simulink model "ADCS_outdated_May3"  (R2018a)
settings: Solver=VariableStepAuto  StartTime=0.0  StopTime=10.0  RelTol=1e-3
undefined symbols (not defined in the file): delta_t, GM_Earth, GM_Moon, GM_Sun, SC
settings Model: Creator=azufall  LastModifiedBy=Hridu

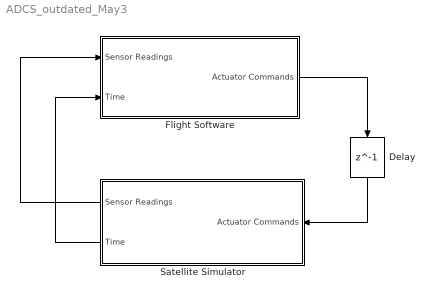
== system ADCS_outdated_May3 ==
  Delay : Delay  DelayLength=1  InitialCondition=0
  Flight Software : Subsystem
  Satellite Simulator : Subsystem
  wires:
  Flight Software/1(Actuator Commands) -> Delay/1
  Satellite Simulator/2(Time) -> Flight Software/2(Time)
  Satellite Simulator/1(Sensor Readings) -> Flight Software/1(Sensor Readings)
  Delay/1 -> Satellite Simulator/1(Actuator Commands)

== system ADCS_outdated_May3/Flight Software ==
  Sensor Readings : Inport
  Time : Inport  Port=2
  Demux : Demux  Outputs=3
  Max thrust : Gain
  Resolution Error : Rounding
  Subsystems : Subsystem
  Actuator Commands : Outport
  wires:
  Subsystems/1(RCS Command) -> Max thrust/1
  Sensor Readings/1 -> Demux/1
  Demux/1 -> Subsystems/1(Gyro)
  Demux/2 -> Subsystems/2(Sun Sensor)
  Demux/3 -> Subsystems/3(Star Tracker)
  Time/1 -> Subsystems/4(Time)
  Max thrust/1 -> Resolution Error/1
  Resolution Error/1 -> Actuator Commands/1

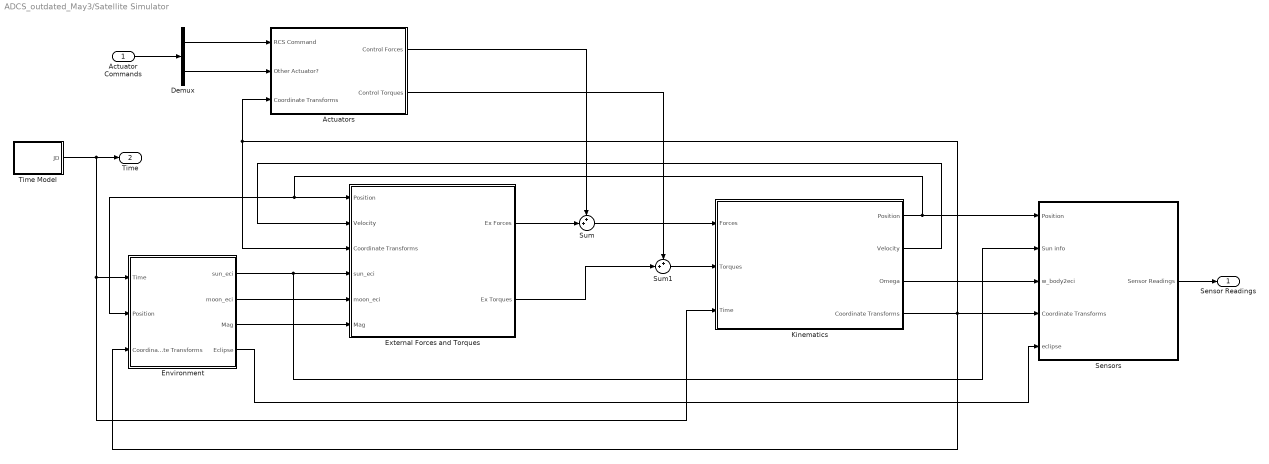
== system ADCS_outdated_May3/Satellite Simulator ==
  Actuator Commands : Inport
  Actuators : Subsystem
  Demux : Demux  Outputs=2
  Environment : Subsystem
  External Forces and Torques : Subsystem
  Kinematics : Subsystem
  Sensors : Subsystem
  Sum : Sum  Inputs=++|
  Sum1 : Sum  Inputs=++|
  Time Model : Subsystem
  Sensor Readings : Outport
  Time : Outport  Port=2
  wires:
  Actuator Commands/1 -> Demux/1
  Demux/1 -> Actuators/1(RCS Command)
  Demux/2 -> Actuators/2(Other Actuator?)
  Kinematics/3(Omega) -> Sensors/3(w_body2eci)
  Sensors/1(Sensor Readings) -> Sensor Readings/1
  Time Model/1(JD) -> Kinematics/3(Time), Environment/1(Time), Time/1
  Environment/1(sun_eci) -> Sensors/2(Sun info), External Forces and Torques/4(sun_eci)
  Environment/2(moon_eci) -> External Forces and Torques/5(moon_eci)
  Environment/3(Mag) -> External Forces and Torques/6(Mag)
  External Forces and Torques/1(Ex Forces) -> Sum/2
  Sum/1 -> Kinematics/1(Forces)
  External Forces and Torques/2(Ex Torques) -> Sum1/2
  Kinematics/2(Velocity) -> External Forces and Torques/2(Velocity)
  Kinematics/4(Coordinate Transforms) -> Environment/3(Coordinate Transforms), Actuators/3(Coordinate Transforms), External Forces and Torques/3(Coordinate Transforms), Sensors/4(Coordinate Transforms)
  Actuators/1(Control Forces) -> Sum/1
  Actuators/2(Control Torques) -> Sum1/1
  Sum1/1 -> Kinematics/2(Torques)
  Kinematics/1(Position) -> Sensors/1(Position), Environment/2(Position), External Forces and Torques/1(Position)
  Environment/4(Eclipse) -> Sensors/5(eclipse)

== system ADCS_outdated_May3/Flight Software/Subsystems ==
  Gyro : Inport
  Sun Sensor : Inport  Port=2
  Star Tracker : Inport  Port=3
  Time : Inport  Port=4
  Mode Selection : Subsystem
  RCS Controller : Subsystem
  Sensor Processing : Subsystem
  RCS Command : Outport
  wires:
  Gyro/1 -> Sensor Processing/1(Gyro_raw)
  Sun Sensor/1 -> Sensor Processing/2(Sun_raw)
  Star Tracker/1 -> Sensor Processing/3(Star_raw)
  Sensor Processing/1(Gyro_filtered) -> RCS Controller/2(Gyro), Mode Selection/1(Gyro)
  Sensor Processing/4(Eclipse) -> Mode Selection/2(Eclipse)
  Time/1 -> RCS Controller/6(Time), Mode Selection/3(Time)
  RCS Controller/1(RCS_Command) -> RCS Command/1
  Mode Selection/2(S/C Mode) -> RCS Controller/1(Mode)
  Mode Selection/1(Controller Gains) -> RCS Controller/5(Gains)
  Sensor Processing/3(Star_filtered) -> RCS Controller/4(Star)
  Sensor Processing/2(Sun_filtered) -> RCS Controller/3(Sun)

== system ADCS_outdated_May3/Satellite Simulator/Actuators ==
  RCS Command : Inport
  Other Actuator? : Inport  Port=2
  Coordinate Transforms : Inport  Port=3
  RCS Model : MATLAB Function  TreatAsAtomicUnit=on
  Control Forces : Outport
  Control Torques : Outport  Port=2
  wires:
  RCS Command/1 -> RCS Model/1(command)
  RCS Model/1(force_body) -> Control Forces/1
  RCS Model/2(torque_body) -> Control Torques/1

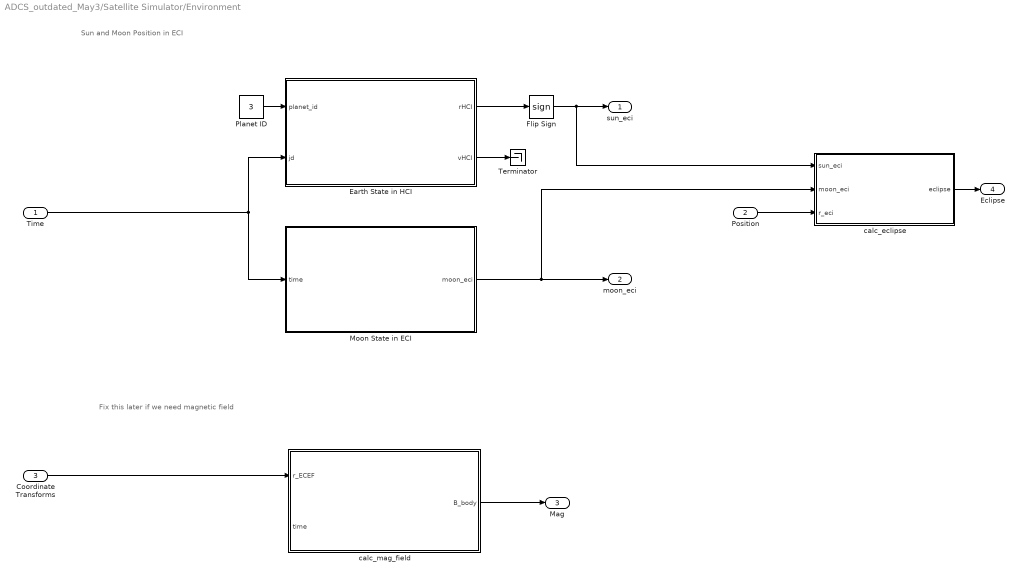
== system ADCS_outdated_May3/Satellite Simulator/Environment ==
  note: Sun and Moon Position in ECI
  note: Fix this later if we need magnetic field
  Time : Inport
  Position : Inport  Port=2
  Coordinate Transforms : Inport  Port=3
  Earth State in HCI : MATLAB Function  TreatAsAtomicUnit=on
  Flip Sign : Signum
  Moon State in ECI : MATLAB Function  TreatAsAtomicUnit=on
  Planet ID : Constant  Value=3
  Terminator : Terminator
  calc_eclipse : MATLAB Function  TreatAsAtomicUnit=on
  calc_mag_field : MATLAB Function  TreatAsAtomicUnit=on
  sun_eci : Outport
  moon_eci : Outport  Port=2
  Mag : Outport  Port=3
  Eclipse : Outport  Port=4
  wires:
  Moon State in ECI/1(moon_eci) -> calc_eclipse/2(moon_eci), moon_eci/1
  calc_mag_field/1(B_body) -> Mag/1
  calc_eclipse/1(eclipse) -> Eclipse/1
  Time/1 -> Earth State in HCI/2(jd), Moon State in ECI/1(time)
  Planet ID/1 -> Earth State in HCI/1(planet_id)
  Earth State in HCI/1(rHCI) -> Flip Sign/1
  Flip Sign/1 -> calc_eclipse/1(sun_eci), sun_eci/1
  Position/1 -> calc_eclipse/3(r_eci)
  Earth State in HCI/2(vHCI) -> Terminator/1
  Coordinate Transforms/1 -> calc_mag_field/1(r_ECEF)

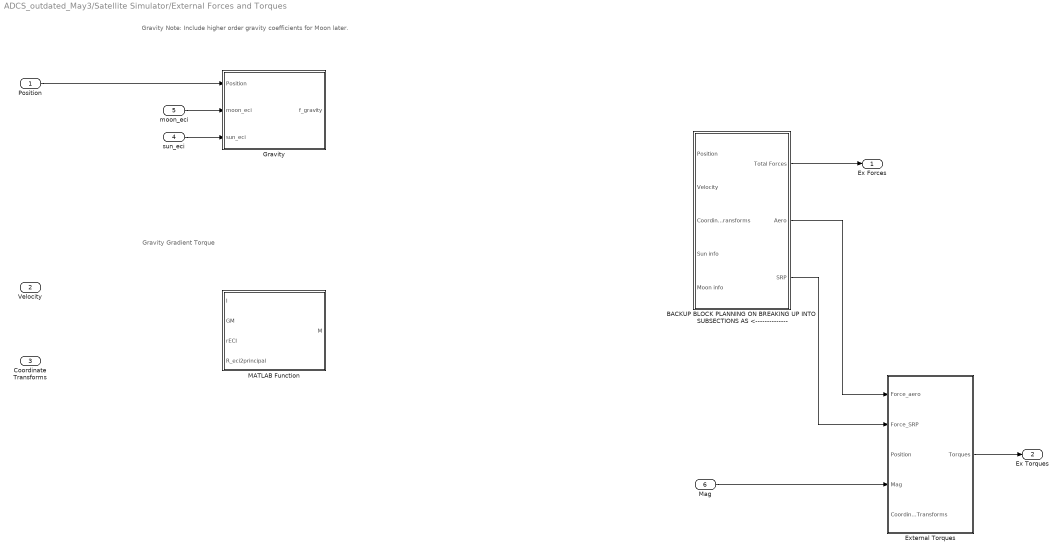
== system ADCS_outdated_May3/Satellite Simulator/External Forces and Torques ==
  note: Gravity Gradient Torque
  note: Gravity
      |
      | Note: Include higher order gravity coefficients for Moon later.
  Position : Inport
  Velocity : Inport  Port=2
  Coordinate Transforms : Inport  Port=3
  sun_eci : Inport  Port=4
  moon_eci : Inport  Port=5
  Mag : Inport  Port=6
  BACKUP BLOCK PLANNING ON BREAKING UP INTO SUBSECTIONS AS <-------------- : Subsystem
  External Torques : Subsystem
  Gravity : Subsystem
  MATLAB Function : MATLAB Function  TreatAsAtomicUnit=on
  Ex Forces : Outport
  Ex Torques : Outport  Port=2
  wires:
  Mag/1 -> External Torques/4(Mag)
  BACKUP BLOCK PLANNING ON BREAKING UP INTO SUBSECTIONS AS <--------------/1(Total Forces) -> Ex Forces/1
  External Torques/1(Torques) -> Ex Torques/1
  BACKUP BLOCK PLANNING ON BREAKING UP INTO SUBSECTIONS AS <--------------/2(Aero) -> External Torques/1(Force_aero)
  BACKUP BLOCK PLANNING ON BREAKING UP INTO SUBSECTIONS AS <--------------/3(SRP) -> External Torques/2(Force_SRP)
  Position/1 -> Gravity/1(Position)
  moon_eci/1 -> Gravity/2(moon_eci)
  sun_eci/1 -> Gravity/3(sun_eci)

== system ADCS_outdated_May3/Satellite Simulator/Kinematics ==
  Forces : Inport
  Torques : Inport  Port=2
  Time : Inport  Port=3
  Calc Coordinate Transforms : Subsystem
  Position Kinematics : Subsystem
  Rotation Kinematics : Subsystem
  TEST POSITION KINEMATICS : Subsystem
  Position : Outport
  Velocity : Outport  Port=2
  Omega : Outport  Port=3
  Coordinate Transforms : Outport  Port=4
  wires:
  Forces/1 -> Position Kinematics/1(a_eci)
  Torques/1 -> Rotation Kinematics/1(tor)
  Rotation Kinematics/2(w) -> Omega/1
  Rotation Kinematics/1(q) -> Calc Coordinate Transforms/4(Attitude)
  Position Kinematics/1(r_eci) -> Position/1, Calc Coordinate Transforms/1(Position)
  Position Kinematics/2(v_eci) -> Velocity/1, Calc Coordinate Transforms/2(Velocity)
  Calc Coordinate Transforms/1(Coordinate Transforms) -> Coordinate Transforms/1
  Time/1 -> Calc Coordinate Transforms/3(Time)

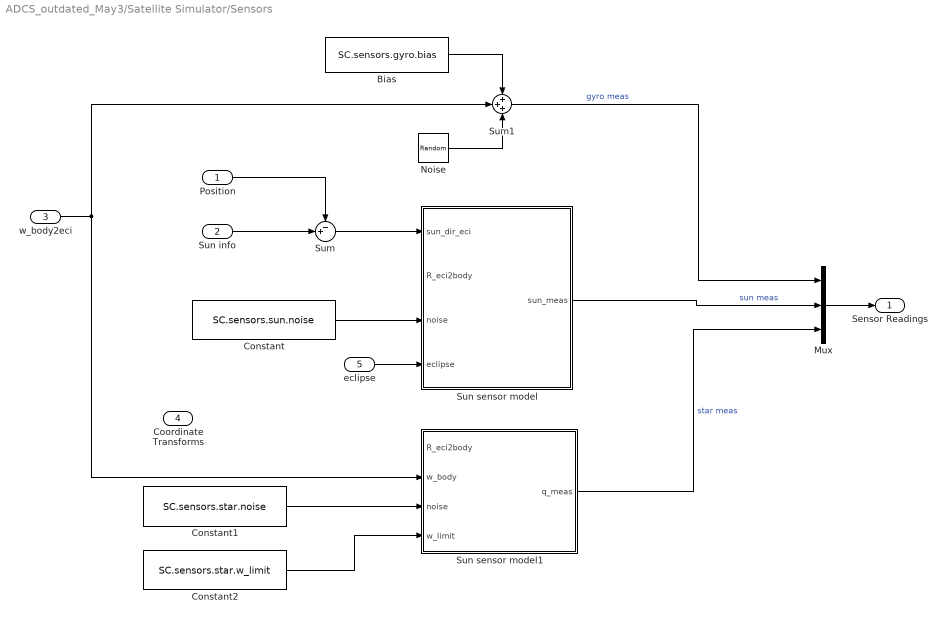
== system ADCS_outdated_May3/Satellite Simulator/Sensors ==
  Position : Inport
  Sun info : Inport  Port=2
  w_body2eci : Inport  Port=3
  Coordinate Transforms : Inport  Port=4
  eclipse : Inport  Port=5
  Bias : Constant  Value=SC.sensors.gyro.bias
  Constant : Constant  Value=SC.sensors.sun.noise
  Constant1 : Constant  Value=SC.sensors.star.noise
  Constant2 : Constant  Value=SC.sensors.star.w_limit
  Mux : Mux  Inputs=3
  Noise : RandomNumber  Variance=SC.sensors.gyro.noise  SampleTime=0.1
  Sum : Sum  Inputs=-+|
  Sum1 : Sum  Inputs=+++
  Sun sensor model : MATLAB Function  TreatAsAtomicUnit=on
  Sun sensor model1 : MATLAB Function  TreatAsAtomicUnit=on
  Sensor Readings : Outport
  wires:
  Mux/1 -> Sensor Readings/1
  Sun sensor model1/1(q_meas) -> Mux/3  "star meas"
  Sun info/1 -> Sum/2
  Position/1 -> Sum/1
  Constant/1 -> Sun sensor model/3(noise)
  Sum/1 -> Sun sensor model/1(sun_dir_eci)
  Sun sensor model/1(sun_meas) -> Mux/2  "sun meas"
  Noise/1 -> Sum1/3
  Bias/1 -> Sum1/1
  w_body2eci/1 -> Sun sensor model1/2(w_body), Sum1/2
  Sum1/1 -> Mux/1  "gyro meas"
  Constant1/1 -> Sun sensor model1/3(noise)
  Constant2/1 -> Sun sensor model1/4(w_limit)
  eclipse/1 -> Sun sensor model/4(eclipse)

== system ADCS_outdated_May3/Satellite Simulator/Time Model ==
  Constant : Constant  Value=SC.initial_state.date  VectorParams1D=off
  Constant1 : Constant  Value=delta_t
  Date2JD : MATLAB Function  TreatAsAtomicUnit=on
  Delay : Delay  DelayLength=1  InitialConditionSource=Input port  InitialCondition=0
      settings: InputPortMap=u0,p4
  Sum : Sum  Inputs=|++
  JD : Outport
  wires:
  Sum/1 -> JD/1, Delay/1
  Constant1/1 -> Sum/2
  Delay/1 -> Sum/1
  Constant/1 -> Date2JD/1(date)
  Date2JD/1(JD) -> Delay/2

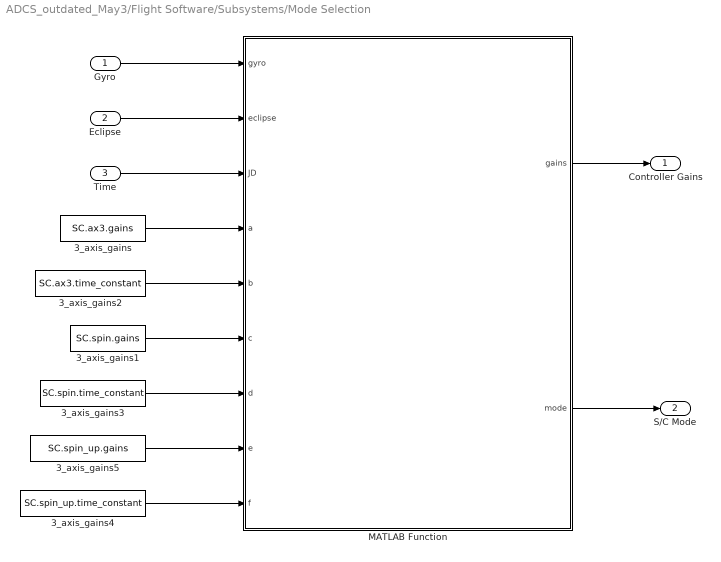
== system ADCS_outdated_May3/Flight Software/Subsystems/Mode Selection ==
  Gyro : Inport
  Eclipse : Inport  Port=2
  Time : Inport  Port=3
  3_axis_gains : Constant  Value=SC.ax3.gains
  3_axis_gains1 : Constant  Value=SC.spin.gains
  3_axis_gains2 : Constant  Value=SC.ax3.time_constant
  3_axis_gains3 : Constant  Value=SC.spin.time_constant
  3_axis_gains4 : Constant  Value=SC.spin_up.time_constant
  3_axis_gains5 : Constant  Value=SC.spin_up.gains
  MATLAB Function : MATLAB Function  TreatAsAtomicUnit=on
  Controller Gains : Outport
  S/C Mode : Outport  Port=2
  wires:
  Time/1 -> MATLAB Function/3(JD)
  Gyro/1 -> MATLAB Function/1(gyro)
  Eclipse/1 -> MATLAB Function/2(eclipse)
  MATLAB Function/1(gains) -> Controller Gains/1
  MATLAB Function/2(mode) -> S/C Mode/1
  3_axis_gains/1 -> MATLAB Function/4(a)
  3_axis_gains2/1 -> MATLAB Function/5(b)
  3_axis_gains1/1 -> MATLAB Function/6(c)
  3_axis_gains3/1 -> MATLAB Function/7(d)
  3_axis_gains5/1 -> MATLAB Function/8(e)
  3_axis_gains4/1 -> MATLAB Function/9(f)

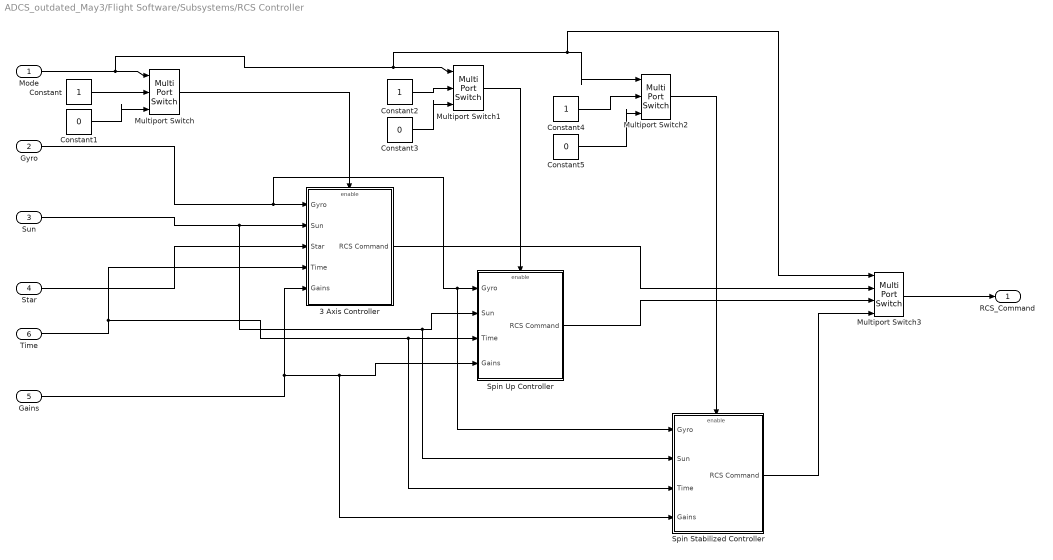
== system ADCS_outdated_May3/Flight Software/Subsystems/RCS Controller ==
  Mode : Inport
  Gyro : Inport  Port=2
  Sun : Inport  Port=3
  Star : Inport  Port=4
  Gains : Inport  Port=5
  Time : Inport  Port=6
  3 Axis Controller : Subsystem  TreatAsAtomicUnit=on
  Constant : Constant
  Constant1 : Constant  Value=0
  Constant2 : Constant
  Constant3 : Constant  Value=0
  Constant4 : Constant
  Constant5 : Constant  Value=0
  Multiport Switch : MultiPortSwitch  Inputs=2
  Multiport Switch1 : MultiPortSwitch  Inputs=2
  Multiport Switch2 : MultiPortSwitch  Inputs=2
  Multiport Switch3 : MultiPortSwitch
  Spin Stabilized Controller : Subsystem  TreatAsAtomicUnit=on
  Spin Up Controller : Subsystem  TreatAsAtomicUnit=on
  RCS_Command : Outport
  wires:
  Multiport Switch/1 -> 3 Axis Controller/Enable
  Multiport Switch1/1 -> Spin Up Controller/Enable
  Multiport Switch2/1 -> Spin Stabilized Controller/Enable
  Mode/1 -> Multiport Switch3/1, Multiport Switch2/1, Multiport Switch1/1, Multiport Switch/1
  Gyro/1 -> Spin Stabilized Controller/1(Gyro), Spin Up Controller/1(Gyro), 3 Axis Controller/1(Gyro)
  Sun/1 -> Spin Stabilized Controller/2(Sun), Spin Up Controller/2(Sun), 3 Axis Controller/2(Sun)
  Star/1 -> 3 Axis Controller/3(Star)
  Time/1 -> Spin Stabilized Controller/3(Time), Spin Up Controller/3(Time), 3 Axis Controller/4(Time)
  Gains/1 -> Spin Stabilized Controller/4(Gains), Spin Up Controller/4(Gains), 3 Axis Controller/5(Gains)
  3 Axis Controller/1(RCS Command) -> Multiport Switch3/2
  Spin Up Controller/1(RCS Command) -> Multiport Switch3/3
  Spin Stabilized Controller/1(RCS Command) -> Multiport Switch3/4
  Multiport Switch3/1 -> RCS_Command/1
  Constant/1 -> Multiport Switch/2
  Constant1/1 -> Multiport Switch/3
  Constant2/1 -> Multiport Switch1/2
  Constant3/1 -> Multiport Switch1/3
  Constant4/1 -> Multiport Switch2/2
  Constant5/1 -> Multiport Switch2/3

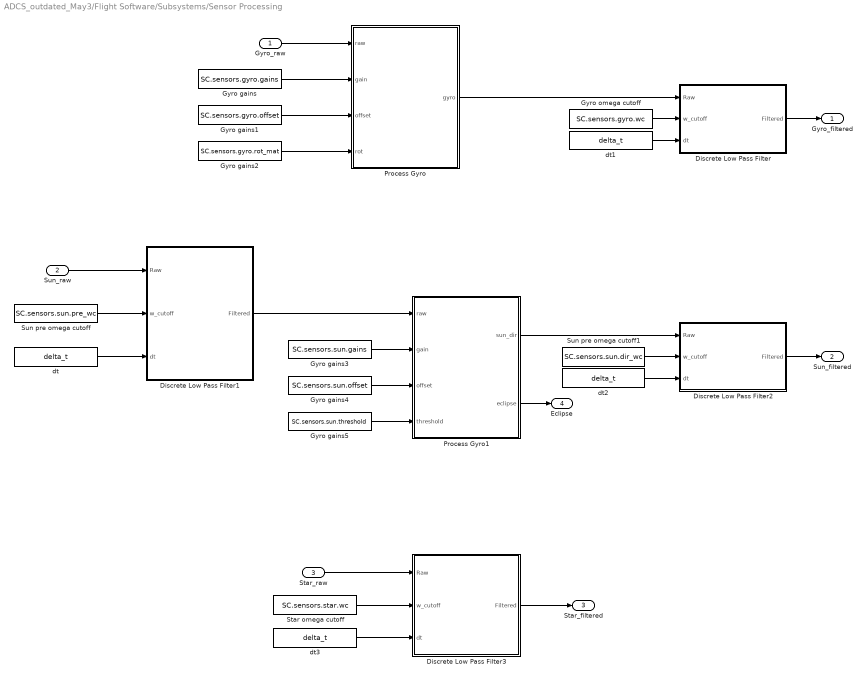
== system ADCS_outdated_May3/Flight Software/Subsystems/Sensor Processing ==
  Gyro_raw : Inport
  Sun_raw : Inport  Port=2
  Star_raw : Inport  Port=3
  Discrete Low Pass Filter : Subsystem
  Discrete Low Pass Filter1 : Subsystem
  Discrete Low Pass Filter2 : Subsystem
  Discrete Low Pass Filter3 : Subsystem
  Gyro gains : Constant  Value=SC.sensors.gyro.gains
  Gyro gains1 : Constant  Value=SC.sensors.gyro.offset
  Gyro gains2 : Constant  Value=SC.sensors.gyro.rot_mat
  Gyro gains3 : Constant  Value=SC.sensors.sun.gains
  Gyro gains4 : Constant  Value=SC.sensors.sun.offset
  Gyro gains5 : Constant  Value=SC.sensors.sun.threshold
  Gyro omega cutoff : Constant  Value=SC.sensors.gyro.wc
  Process Gyro : MATLAB Function  TreatAsAtomicUnit=on
  Process Gyro1 : MATLAB Function  TreatAsAtomicUnit=on
  Star omega cutoff : Constant  Value=SC.sensors.star.wc
  Sun pre omega cutoff : Constant  Value=SC.sensors.sun.pre_wc
  Sun pre omega cutoff1 : Constant  Value=SC.sensors.sun.dir_wc
  dt{,1..3} (4 alike) : Constant  Value=delta_t
  Gyro_filtered : Outport
  Sun_filtered : Outport  Port=2
  Star_filtered : Outport  Port=3
  Eclipse : Outport  Port=4
  wires:
  Gyro_raw/1 -> Process Gyro/1(raw)
  Gyro gains/1 -> Process Gyro/2(gain)
  Gyro gains1/1 -> Process Gyro/3(offset)
  Gyro gains2/1 -> Process Gyro/4(rot)
  Discrete Low Pass Filter/1(Filtered) -> Gyro_filtered/1
  Process Gyro/1(gyro) -> Discrete Low Pass Filter/1(Raw)
  Gyro omega cutoff/1 -> Discrete Low Pass Filter/2(w_cutoff)
  dt1/1 -> Discrete Low Pass Filter/3(dt)
  Sun_raw/1 -> Discrete Low Pass Filter1/1(Raw)
  Discrete Low Pass Filter1/1(Filtered) -> Process Gyro1/1(raw)
  Discrete Low Pass Filter2/1(Filtered) -> Sun_filtered/1
  Process Gyro1/1(sun_dir) -> Discrete Low Pass Filter2/1(Raw)
  Process Gyro1/2(eclipse) -> Eclipse/1
  Sun pre omega cutoff/1 -> Discrete Low Pass Filter1/2(w_cutoff)
  dt/1 -> Discrete Low Pass Filter1/3(dt)
  Gyro gains3/1 -> Process Gyro1/2(gain)
  Gyro gains4/1 -> Process Gyro1/3(offset)
  Gyro gains5/1 -> Process Gyro1/4(threshold)
  Sun pre omega cutoff1/1 -> Discrete Low Pass Filter2/2(w_cutoff)
  dt2/1 -> Discrete Low Pass Filter2/3(dt)
  Star_raw/1 -> Discrete Low Pass Filter3/1(Raw)
  Discrete Low Pass Filter3/1(Filtered) -> Star_filtered/1
  Star omega cutoff/1 -> Discrete Low Pass Filter3/2(w_cutoff)
  dt3/1 -> Discrete Low Pass Filter3/3(dt)

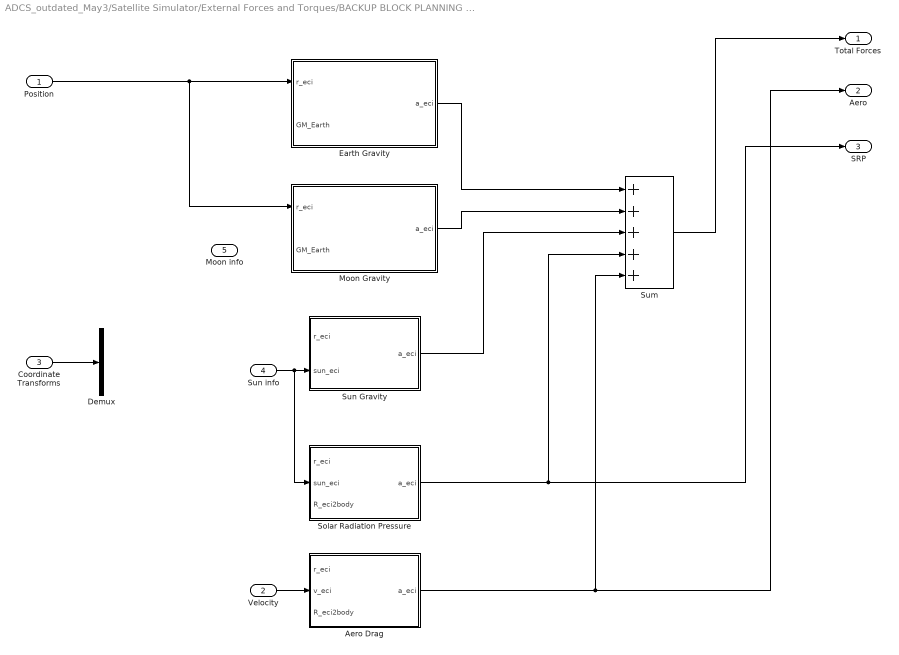
== system ADCS_outdated_May3/Satellite Simulator/External Forces and Torques/BACKUP BLOCK PLANNING ON BREAKING UP INTO SUBSECTIONS AS <-------------- ==
  Position : Inport
  Velocity : Inport  Port=2
  Coordinate Transforms : Inport  Port=3
  Sun info : Inport  Port=4
  Moon info : Inport  Port=5
  Aero Drag : MATLAB Function  TreatAsAtomicUnit=on
  Demux : Demux
  Earth Gravity : MATLAB Function  TreatAsAtomicUnit=on
  Moon Gravity : MATLAB Function  TreatAsAtomicUnit=on
  Solar Radiation Pressure : MATLAB Function  TreatAsAtomicUnit=on
  Sum : Sum  Inputs=+++++
  Sun Gravity : MATLAB Function  TreatAsAtomicUnit=on
  Total Forces : Outport
  Aero : Outport  Port=2
  SRP : Outport  Port=3
  wires:
  Position/1 -> Moon Gravity/1(r_eci), Earth Gravity/1(r_eci)
  Sun info/1 -> Solar Radiation Pressure/2(sun_eci), Sun Gravity/2(sun_eci)
  Solar Radiation Pressure/1(a_eci) -> Sum/4, SRP/1
  Aero Drag/1(a_eci) -> Sum/5, Aero/1
  Sum/1 -> Total Forces/1
  Earth Gravity/1(a_eci) -> Sum/1
  Sun Gravity/1(a_eci) -> Sum/3
  Velocity/1 -> Aero Drag/2(v_eci)
  Coordinate Transforms/1 -> Demux/1
  Moon Gravity/1(a_eci) -> Sum/2

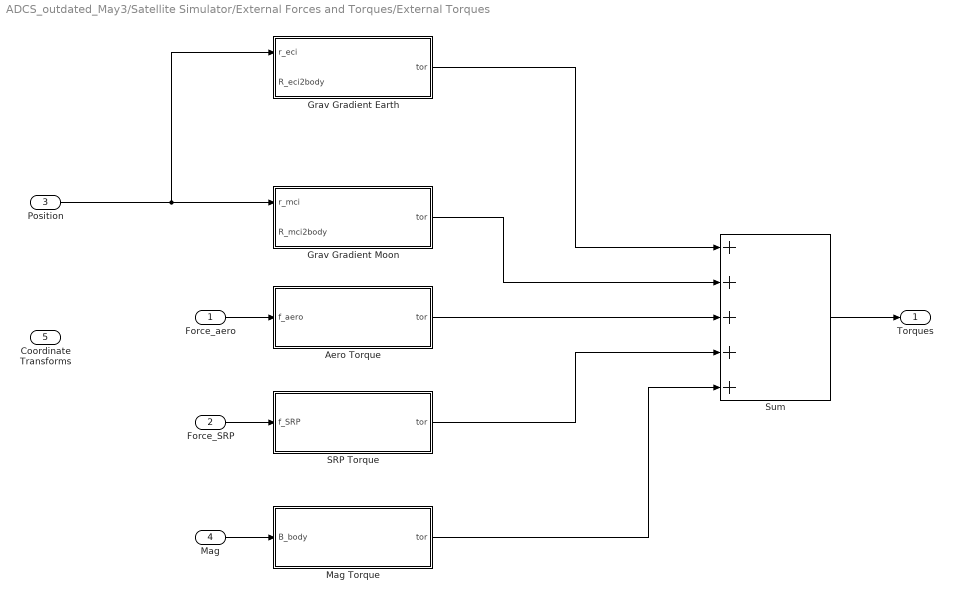
== system ADCS_outdated_May3/Satellite Simulator/External Forces and Torques/External Torques ==
  Force_aero : Inport
  Force_SRP : Inport  Port=2
  Position : Inport  Port=3
  Mag : Inport  Port=4
  Coordinate Transforms : Inport  Port=5
  Aero Torque : MATLAB Function  TreatAsAtomicUnit=on
  Grav Gradient Earth : MATLAB Function  TreatAsAtomicUnit=on
  Grav Gradient Moon : MATLAB Function  TreatAsAtomicUnit=on
  Mag Torque : MATLAB Function  TreatAsAtomicUnit=on
  SRP Torque : MATLAB Function  TreatAsAtomicUnit=on
  Sum : Sum  Inputs=5
  Torques : Outport
  wires:
  Position/1 -> Grav Gradient Moon/1(r_mci), Grav Gradient Earth/1(r_eci)
  Sum/1 -> Torques/1
  Grav Gradient Earth/1(tor) -> Sum/1
  Grav Gradient Moon/1(tor) -> Sum/2
  Aero Torque/1(tor) -> Sum/3
  Force_aero/1 -> Aero Torque/1(f_aero)
  Force_SRP/1 -> SRP Torque/1(f_SRP)
  SRP Torque/1(tor) -> Sum/4
  Mag Torque/1(tor) -> Sum/5
  Mag/1 -> Mag Torque/1(B_body)

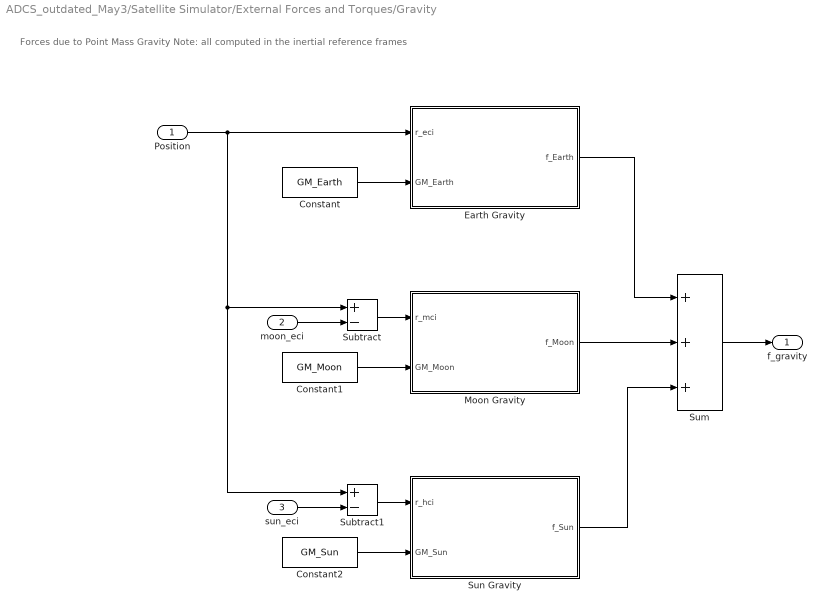
== system ADCS_outdated_May3/Satellite Simulator/External Forces and Torques/Gravity ==
  note: Forces due to Point Mass Gravity
      |
      | Note: all computed in the inertial reference frames
  Position : Inport
  moon_eci : Inport  Port=2
  sun_eci : Inport  Port=3
  Constant : Constant  Value=GM_Earth
  Constant1 : Constant  Value=GM_Moon
  Constant2 : Constant  Value=GM_Sun
  Earth Gravity : MATLAB Function  TreatAsAtomicUnit=on
  Moon Gravity : MATLAB Function  TreatAsAtomicUnit=on
  Subtract : Sum  Inputs=+-
  Subtract1 : Sum  Inputs=+-
  Sum : Sum  Inputs=+++
  Sun Gravity : MATLAB Function  TreatAsAtomicUnit=on
  f_gravity : Outport
  wires:
  Position/1 -> Earth Gravity/1(r_eci), Subtract/1, Subtract1/1
  Sum/1 -> f_gravity/1
  Earth Gravity/1(f_Earth) -> Sum/1
  Sun Gravity/1(f_Sun) -> Sum/3
  Moon Gravity/1(f_Moon) -> Sum/2
  moon_eci/1 -> Subtract/2
  Subtract/1 -> Moon Gravity/1(r_mci)
  Subtract1/1 -> Sun Gravity/1(r_hci)
  sun_eci/1 -> Subtract1/2
  Constant/1 -> Earth Gravity/2(GM_Earth)
  Constant1/1 -> Moon Gravity/2(GM_Moon)
  Constant2/1 -> Sun Gravity/2(GM_Sun)

== system ADCS_outdated_May3/Satellite Simulator/Kinematics/Calc Coordinate Transforms ==
  Position : Inport
  Velocity : Inport  Port=2
  Time : Inport  Port=3
  Attitude : Inport  Port=4
  Mux : Mux
  Coordinate Transforms : Outport
  wires:
  Mux/1 -> Coordinate Transforms/1

== system ADCS_outdated_May3/Satellite Simulator/Kinematics/Position Kinematics ==
  a_eci : Inport
  3 DOF Kinematics : MATLAB Function  TreatAsAtomicUnit=on
  Constant : Constant  Value=SC.initial_state.r_eci
  Constant1 : Constant  Value=SC.initial_state.v_eci
  Constant2 : Constant  Value=delta_t
  Delay : Delay  DelayLength=1  InitialConditionSource=Input port  InitialCondition=0
      settings: InputPortMap=u0,p4
  Delay1 : Delay  DelayLength=1  InitialConditionSource=Input port  InitialCondition=0
      settings: InputPortMap=u0,p4
  r_eci : Outport
  v_eci : Outport  Port=2
  wires:
  a_eci/1 -> 3 DOF Kinematics/3(a_eci)
  3 DOF Kinematics/1(r_eci) -> Delay/1, r_eci/1
  3 DOF Kinematics/2(v_eci) -> Delay1/1, v_eci/1
  Delay/1 -> 3 DOF Kinematics/1(r_eci_i)
  Delay1/1 -> 3 DOF Kinematics/2(v_eci_i)
  Constant/1 -> Delay/2
  Constant1/1 -> Delay1/2
  Constant2/1 -> 3 DOF Kinematics/4(dt)

== system ADCS_outdated_May3/Satellite Simulator/Kinematics/Rotation Kinematics ==
  tor : Inport
  Constant : Constant  Value=SC.initial_state.q
  Constant1 : Constant  Value=SC.initial_state.w
  Constant2 : Constant  Value=delta_t
  Delay : Delay  DelayLength=1  InitialConditionSource=Input port  InitialCondition=0
      settings: InputPortMap=u0,p4
  Delay1 : Delay  DelayLength=1  InitialConditionSource=Input port  InitialCondition=0
      settings: InputPortMap=u0,p4
  Euler Equations : MATLAB Function  TreatAsAtomicUnit=on
  q : Outport
  w : Outport  Port=2
  wires:
  tor/1 -> Euler Equations/3(tor)
  Euler Equations/1(q) -> Delay/1, q/1
  Delay/1 -> Euler Equations/1(q_i)
  Delay1/1 -> Euler Equations/2(w_i)
  Constant/1 -> Delay/2
  Constant1/1 -> Delay1/2
  Constant2/1 -> Euler Equations/4(dt)
  Euler Equations/2(w) -> Delay1/1, w/1

== system ADCS_outdated_May3/Satellite Simulator/Kinematics/TEST POSITION KINEMATICS ==
  a_eci : Inport
  Constant3 : Constant  Value=SC.initial_state.r_eci
  Constant4 : Constant  Value=SC.initial_state.v_eci
  Integrator : Integrator  InitialConditionSource=external
  Integrator1 : Integrator  InitialConditionSource=external
  r_eci : Outport
  v_eci : Outport  Port=2
  wires:
  Constant4/1 -> Integrator/2
  a_eci/1 -> Integrator/1
  Integrator/1 -> v_eci/1, Integrator1/1
  Constant3/1 -> Integrator1/2
  Integrator1/1 -> r_eci/1

== system ADCS_outdated_May3/Flight Software/Subsystems/RCS Controller/3 Axis Controller ==
  Gyro : Inport
  Sun : Inport  Port=2
  Star : Inport  Port=3
  Time : Inport  Port=4
  Gains : Inport  Port=5
  Enable : EnablePort
  RCS Command : Outport
  wires:
  Gyro/1 -> RCS Command/1

== system ADCS_outdated_May3/Flight Software/Subsystems/RCS Controller/Spin Stabilized Controller ==
  Gyro : Inport
  Sun : Inport  Port=2
  Time : Inport  Port=3
  Gains : Inport  Port=4
  Enable : EnablePort
  RCS Command : Outport
  wires:
  Gyro/1 -> RCS Command/1

== system ADCS_outdated_May3/Flight Software/Subsystems/RCS Controller/Spin Up Controller ==
  Gyro : Inport
  Sun : Inport  Port=2
  Time : Inport  Port=3
  Gains : Inport  Port=4
  Enable : EnablePort
  RCS Command : Outport
  wires:
  Gyro/1 -> RCS Command/1

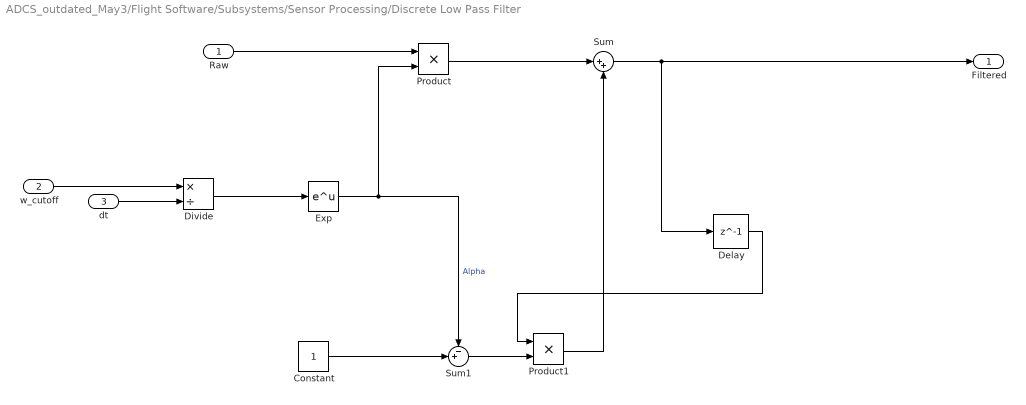
== system ADCS_outdated_May3/Flight Software/Subsystems/Sensor Processing/Discrete Low Pass Filter ==
  Raw : Inport
  w_cutoff : Inport  Port=2
  dt : Inport  Port=3
  Constant : Constant
  Delay : Delay  DelayLength=1  InitialCondition=0
  Divide : Product  Inputs=*/
  Exp : Math  SaturateOnIntegerOverflow=on
  Product : Product
  Product1 : Product
  Sum : Sum  Inputs=|++
  Sum1 : Sum  Inputs=-+|
  Filtered : Outport
  wires:
  w_cutoff/1 -> Divide/1
  dt/1 -> Divide/2
  Divide/1 -> Exp/1
  Exp/1 -> Sum1/1, Product/2  "Alpha"
  Raw/1 -> Product/1
  Product/1 -> Sum/1
  Sum/1 -> Delay/1, Filtered/1
  Constant/1 -> Sum1/2
  Sum1/1 -> Product1/2
  Delay/1 -> Product1/1
  Product1/1 -> Sum/2

== system ADCS_outdated_May3/Flight Software/Subsystems/Sensor Processing/Discrete Low Pass Filter1 ==
  Raw : Inport
  w_cutoff : Inport  Port=2
  dt : Inport  Port=3
  Constant : Constant
  Delay : Delay  DelayLength=1  InitialCondition=0
  Divide : Product  Inputs=*/
  Exp : Math  SaturateOnIntegerOverflow=on
  Product : Product
  Product1 : Product
  Sum : Sum  Inputs=|++
  Sum1 : Sum  Inputs=-+|
  Filtered : Outport
  wires:
  w_cutoff/1 -> Divide/1
  dt/1 -> Divide/2
  Divide/1 -> Exp/1
  Exp/1 -> Sum1/1, Product/2  "Alpha"
  Raw/1 -> Product/1
  Product/1 -> Sum/1
  Sum/1 -> Delay/1, Filtered/1
  Constant/1 -> Sum1/2
  Sum1/1 -> Product1/2
  Delay/1 -> Product1/1
  Product1/1 -> Sum/2

== system ADCS_outdated_May3/Flight Software/Subsystems/Sensor Processing/Discrete Low Pass Filter2 ==
  Raw : Inport
  w_cutoff : Inport  Port=2
  dt : Inport  Port=3
  Constant : Constant
  Delay : Delay  DelayLength=1  InitialCondition=0
  Divide : Product  Inputs=*/
  Exp : Math  SaturateOnIntegerOverflow=on
  Product : Product
  Product1 : Product
  Sum : Sum  Inputs=|++
  Sum1 : Sum  Inputs=-+|
  Filtered : Outport
  wires:
  w_cutoff/1 -> Divide/1
  dt/1 -> Divide/2
  Divide/1 -> Exp/1
  Exp/1 -> Sum1/1, Product/2  "Alpha"
  Raw/1 -> Product/1
  Product/1 -> Sum/1
  Sum/1 -> Delay/1, Filtered/1
  Constant/1 -> Sum1/2
  Sum1/1 -> Product1/2
  Delay/1 -> Product1/1
  Product1/1 -> Sum/2

== system ADCS_outdated_May3/Flight Software/Subsystems/Sensor Processing/Discrete Low Pass Filter3 ==
  Raw : Inport
  w_cutoff : Inport  Port=2
  dt : Inport  Port=3
  Constant : Constant
  Delay : Delay  DelayLength=1  InitialCondition=0
  Divide : Product  Inputs=*/
  Exp : Math  SaturateOnIntegerOverflow=on
  Product : Product
  Product1 : Product
  Sum : Sum  Inputs=|++
  Sum1 : Sum  Inputs=-+|
  Filtered : Outport
  wires:
  w_cutoff/1 -> Divide/1
  dt/1 -> Divide/2
  Divide/1 -> Exp/1
  Exp/1 -> Sum1/1, Product/2  "Alpha"
  Raw/1 -> Product/1
  Product/1 -> Sum/1
  Sum/1 -> Delay/1, Filtered/1
  Constant/1 -> Sum1/2
  Sum1/1 -> Product1/2
  Delay/1 -> Product1/1
  Product1/1 -> Sum/2

== matlab function ADCS_outdated_May3/Flight Software/Subsystems/Sensor Processing/Process Gyro ==
  data: raw input; gyro output; gain input; offset input; rot input
function gyro = process_gyro(raw, gain, offset, rot)

temp = rot * raw;
gyro = gain * (temp - offset);

== matlab function ADCS_outdated_May3/Flight Software/Subsystems/Mode Selection/MATLAB Function ==
  data: gyro input; gains output; eclipse input; JD input; mode output; a input; b input; c input; d input; e input; f input
function [gains, mode]  = Mode_Logic(gyro, eclipse, JD, a,b,c,d,e,f)

gains = [1;1;1];
mode = 1;

%switch case, determine what part of mission we are in

== matlab function ADCS_outdated_May3/Flight Software/Subsystems/Sensor Processing/Process Gyro1 ==
  data: raw input; sun_dir output; gain input; offset input; eclipse output; threshold input
function [sun_dir, eclipse] = process_sun(raw, gain, offset, threshold)
n = length(raw); %number of sun sensors
sun = zeros(n,1);
for i=1:length(raw)
    sun(i) = gain(i) * (raw(i) - offset(i));
end

%discuss advantages of different ways of turning sun measurements to direction
sun_x = sun(1)-sun(2);
sun_y = sun(3)-sun(4);
sun_z = sun(5)-sun(6);

sun_dir = [sun_x; sun_y; sun_z];
sun_dir = sun_dir/norm(sun_dir);

eclipse = 0;
if (sum(abs(sun < threshold)))
    eclipse = 1;
end

== matlab function ADCS_outdated_May3/Satellite Simulator/External Forces and Torques/MATLAB Function ==
  data: I input; M output; GM input; rECI input; R_eci2principal input
function M = gravityGradient(I, GM, rECI, R_eci2principal)
% Expressed in principal axes. The c vector is the position vector of the
% satellite expressed in principal axes.

R = norm(rECI);
c = R_eci2principal*rECI;

Ix = I(1,1);
Iy = I(2,2);
Iz = I(3,3);
cx = c(1);
cy = c(2);
cz = c(3);

M = zeros(3,1);
M(1) = 3*GM/R^3 * (Iz - Iy)*cy*cz;
M(2) = 3*GM/R^3 * (Ix - Iz)*cz*cx;
M(3) = 3*GM/R^3 * (Iy - Ix)*cx*cy;
end

== matlab function ADCS_outdated_May3/Satellite Simulator/External Forces and Torques/Gravity/Earth Gravity ==
  data: r_eci input; f_Earth output; GM_Earth input
function f_Earth = accelPointMass(r_eci, GM_Earth)
f_Earth = -GM_Earth*r_eci./norm(r_eci)^3;
end

== matlab function ADCS_outdated_May3/Satellite Simulator/External Forces and Torques/Gravity/Moon Gravity ==
  data: r_mci input; f_Moon output; GM_Moon input
function f_Moon = accelPointMass(r_mci, GM_Moon)
f_Moon = -GM_Moon*r_mci./norm(r_mci)^3;
end

== matlab function ADCS_outdated_May3/Satellite Simulator/External Forces and Torques/Gravity/Sun Gravity ==
  data: r_hci input; f_Sun output; GM_Sun input
function f_Sun = accelPointMass(r_hci, GM_Sun)
f_Sun = -GM_Sun*r_hci./norm(r_hci)^3;
end

== matlab function ADCS_outdated_May3/Satellite Simulator/Actuators/RCS Model ==
  data: command input; force_body output; torque_body output
function [force_body, torque_body] = fcn(command)

force_body = [0;0;0];
torque_body = [0;0;0];

== matlab function ADCS_outdated_May3/Satellite Simulator/Environment/Earth State in HCI ==
  data: planet_id input; rHCI output; jd input; vHCI output
function [rHCI, vHCI] = AA279planet_state(planet_id, jd)
% Returns heliocentric position and velocity of planet at given time
%
% AA279 Function Library
% Last modified: 22 April 2016 by Andrew K. Barrows

% Physical constants from http://ssd.jpl.nasa.gov/horizons.cgi  Feb 2014
km_per_au = 149597870.700; % [km/AU]
musun     = 1.3271244004193938e11; % [km^3/sec^2]

% Get data for selected planet
[j2000_elements, rates] = AA279j2000_planetary_elements(planet_id);

% Find elements at given time
elements = j2000_elements + rates*(jd - 2451545)/36525;

a = elements(1)*km_per_au; % semi-major axis
ecc = elements(2); % eccentricity

p = a*(1 - ecc*ecc); % [km]

inc = elements(3); % [deg] inclination (assume stays in [-90 +90] range)

LAN = elements(4); % [deg] longitude of ascending node
while LAN >= 360.0
    LAN = LAN - 360.0; 
end
while LAN < 0.0
    LAN = LAN + 360.0;
end

omega_bar = elements(5); % [deg] longitude of perihelion
while omega_bar >= 360.0
    omega_bar = omega_bar - 360.0; 
end
while omega_bar < 0.0
    omega_bar = omega_bar + 360.0;
end

L = elements(6); % [deg] mean longitude
while L >= 360.0
    L = L - 360.0; 
end
while L < 0.0
    L = L + 360.0;
end  

omega = omega_bar - LAN; % [deg] argument of perihelion
while omega >= 360.0
    omega = omega - 360.0; 
end
while omega < 0.0
    omega = omega + 360.0;
end 

M = L - omega_bar; % [deg] mean anomaly
while M >= 360.0
    M = M - 360.0; 
end
while M < 0.0
    M = M + 360.0;
end 

% Find eccentric anomaly by solving Kepler's equation
E = AA279solve_kepler(M*pi/180, ecc, 1e-10); % [rad]

% Find position and velocity of planet in perifocal coordinates
sinnu = (sin(E)*sqrt(1.0-ecc*ecc))/(1.0-ecc*cos(E));
cosnu = (cos(E)-ecc)/(1.0-ecc*cos(E));
r = p/(1.0+ecc*cosnu); % Trajectory Equation
O_r_P__peri = [r*cosnu; r*sinnu; 0.0];
sqrtmuoverp = sqrt(musun/p);
peri_v_P__peri = [-sqrtmuoverp*sinnu; sqrtmuoverp*(ecc+cosnu); 0.0];
      
% Convert perifocal coordinates to heliocentric coordinates
sinLAN = sin(LAN*pi/180.0);
cosLAN = cos(LAN*pi/180.0);
sininc = sin(inc*pi/180.0);
cosinc = cos(inc*pi/180.0);
sinomega = sin(omega*pi/180.0);
cosomega = cos(omega*pi/180.0);
heli_C_peri = [+cosLAN*cosomega-sinLAN*sinomega*cosinc ...
                  -cosLAN*sinomega-sinLAN*cosomega*cosinc ...
                      +sinLAN*sininc; ...
              +sinLAN*cosomega+cosLAN*sinomega*cosinc ...
                  -sinLAN*sinomega+cosLAN*cosomega*cosinc ...
                      -cosLAN*sininc; ...       
              +sinomega*sininc ...
                  +cosomega*sininc ...
                      +cosinc];
rHCI = heli_C_peri*O_r_P__peri;
vHCI = heli_C_peri*peri_v_P__peri; % because heli_omega_peri = 0

end % terminates MATLAB function


function [E] = AA279solve_kepler(M, e, tol)
% Solves Kepler's Equation using Newton's method
%
% AA279 Function Library
% Last modified: 22 April 2016 by Andrew K. Barrows
%
% E    Eccentric Anomaly [rad]
% M    Mean Anomaly [rad]
% e    eccentricity [dimensionless]
% tol  tolerance value on E for stopping iteration [rad]

E   = (pi+M)/2;  % initial guess
err = tol + 1.0; % ensures at least one iteration will take place

% Iterate using Newton's method
while err >= tol
    Enew = E + (M-E+e*sin(E))/(1-e*cos(E));
    err = abs(Enew-E);
    E = Enew;
end

end % terminates MATLAB function

function [elements, rates] = AA279j2000_planetary_elements(planet_id)
% Returns a planet's J2000 orbital elements and centennial rates
%
% AA279 Function Library
% Last modified: 22 April 2016 by Andrew K. Barrows
%
% Adapted from Orbital Mechanics for Engineering Students by Howard Curtis
% 
% Data valid for the period 1800 AD - 2050 AD
% Source of data: http://ssd.jpl.nasa.gov/?planet_pos
%
% planet_id: 1 through 9, for Mercury through Pluto
%  
% elements:  row vector of J2000 orbital elements for "planet_id"
%                a             semimajor axis [AU]
%                e             eccentricity
%                i             inclination [deg]
%                OMEGA         longitude of the ascending node [deg]
%                omega_bar     longitude of perihelion [deg]
%                L             mean longitude [deg]                   
%                                         
% rates:     row vector of J2000 centennial rates for "planet_id"    
%                a_dot         [AU/cty] (AU per century)
%                e_dot         [1/cty]
%                i_dot         [deg/cty]
%                OMEGA_dot     [deg/cty]
%                omega_bar_dot [deg/cty]
%                L_dot         [deg/cty]
%
%     a           e          i          OMEGA      omega_bar        L

J2000_elements = ...
[0.38709927  0.20563593  7.00497902  48.33076593  77.45779628  252.25032350
 0.72333566  0.00677672  3.39467605  76.67984255 131.60246718  181.97909950 
 1.00000261  0.01671123 -0.00001531   0.0        102.93768193  100.46457166 
 1.52371034  0.09339410  1.84969142  49.55953891 -23.94362959 	-4.55343205
 5.20288700  0.04838624  1.30439695 100.47390909  14.72847983 	34.39644501
 9.53667594  0.05386179  2.48599187 113.66242448  92.59887831 	49.95424423
19.18916464  0.04725744  0.77263783  74.01692503 170.95427630  313.23810451
30.06992276  0.00859048  1.77004347 131.78422574  44.96476227  -55.12002969 
39.48211675  0.24882730 17.14001206 110.30393684 224.06891629  238.92903833];

centennial_rates = ... 
[0.00000037  0.00001906 -0.00594749 -0.12534081  0.16047689  149472.67411175 
 0.00000390 -0.00004107 -0.00078890 -0.27769418  0.00268329	  58517.81538729  
 0.00000562 -0.00004392 -0.01294668  0.0         0.32327364   35999.37244981  
 0.0001847 	 0.00007882 -0.00813131 -0.29257343  0.44441088   19140.30268499  
-0.00011607 -0.00013253 -0.00183714  0.20469106	 0.21252668    3034.74612775 
-0.00125060 -0.00050991  0.00193609 -0.28867794 -0.41897216    1222.49362201
-0.00196176 -0.00004397 -0.00242939  0.04240589  0.40805281 	428.48202785 
 0.00026291  0.00005105  0.00035372 -0.00508664 -0.32241464 	218.45945325 
-0.00031596  0.00005170  0.00004818 -0.01183482 -0.04062942 	145.20780515]; 
 
elements = J2000_elements(planet_id, :);
rates = centennial_rates(planet_id, :);
end % terminates MATLAB function

== matlab function ADCS_outdated_May3/Satellite Simulator/Environment/Moon State in ECI ==
  data: time input; moon_eci output
function moon_eci = fcn(time)

moon_eci = [0;0;0];
end

== matlab function ADCS_outdated_May3/Satellite Simulator/Environment/calc_eclipse ==
  data: sun_eci input; eclipse output; moon_eci input; r_eci input
function eclipse = fcn(sun_eci, moon_eci, r_eci)

eclipse = 0;

if( dot(r_eci, sun_eci) < 0.1)
    eclipse = 1;
end

== matlab function ADCS_outdated_May3/Satellite Simulator/Environment/calc_mag_field ==
  data: r_ECEF input; B_body output; time input
function B_body = fcn(r_ECEF, time)

B_body = r_ECEF;

== matlab function ADCS_outdated_May3/Satellite Simulator/External Forces and Torques/BACKUP BLOCK PLANNING ON BREAKING UP INTO SUBSECTIONS AS <--------------/Aero Drag ==
  data: r_eci input; a_eci output; v_eci input; R_eci2body input
function a_eci = fcn(r_eci, v_eci, R_eci2body)

a_eci = r_eci;

== matlab function ADCS_outdated_May3/Satellite Simulator/External Forces and Torques/BACKUP BLOCK PLANNING ON BREAKING UP INTO SUBSECTIONS AS <--------------/Earth Gravity ==
  data: r_eci input; a_eci output; GM_Earth input
function a_eci = accelPointMass(r_eci, GM_Earth)
a_eci = -GM_Earth*r_eci./norm(r_eci)^3;
end

== matlab function ADCS_outdated_May3/Satellite Simulator/External Forces and Torques/BACKUP BLOCK PLANNING ON BREAKING UP INTO SUBSECTIONS AS <--------------/Moon Gravity ==
  data: r_eci input; a_eci output; GM_Earth input
function a_eci = accelPointMass(r_eci, GM_Earth)
a_eci = -GM_Earth*r_eci./norm(r_eci)^3;
end

== matlab function ADCS_outdated_May3/Satellite Simulator/External Forces and Torques/BACKUP BLOCK PLANNING ON BREAKING UP INTO SUBSECTIONS AS <--------------/Solar Radiation Pressure ==
  data: r_eci input; a_eci output; sun_eci input; R_eci2body input
function a_eci = fcn(r_eci, sun_eci, R_eci2body)

a_eci = r_eci;

== matlab function ADCS_outdated_May3/Satellite Simulator/External Forces and Torques/BACKUP BLOCK PLANNING ON BREAKING UP INTO SUBSECTIONS AS <--------------/Sun Gravity ==
  data: r_eci input; a_eci output; sun_eci input
function a_eci = fcn(r_eci, sun_eci)

a_eci = r_eci;

== matlab function ADCS_outdated_May3/Satellite Simulator/External Forces and Torques/External Torques/Aero Torque ==
  data: f_aero input; tor output
function tor = fcn(f_aero)

tor = f_aero;

== matlab function ADCS_outdated_May3/Satellite Simulator/External Forces and Torques/External Torques/Grav Gradient Earth ==
  data: r_eci input; tor output; R_eci2body input
function tor = fcn(r_eci, R_eci2body)

tor = r_eci;

== matlab function ADCS_outdated_May3/Satellite Simulator/External Forces and Torques/External Torques/Grav Gradient Moon ==
  data: r_mci input; tor output; R_mci2body input
function tor = fcn(r_mci, R_mci2body)

tor = r_mci;

== matlab function ADCS_outdated_May3/Satellite Simulator/External Forces and Torques/External Torques/Mag Torque ==
  data: B_body input; tor output
function tor = fcn(B_body)

tor = B_body;

== matlab function ADCS_outdated_May3/Satellite Simulator/External Forces and Torques/External Torques/SRP Torque ==
  data: f_SRP input; tor output
function tor = fcn(f_SRP)

tor = f_SRP;

== matlab function ADCS_outdated_May3/Satellite Simulator/Kinematics/Position Kinematics/3 DOF Kinematics ==
  data: r_eci_i input; r_eci output; v_eci_i input; a_eci input; dt input; v_eci output
function [r_eci, v_eci] = fcn(r_eci_i, v_eci_i, a_eci, dt)

r_eci = r_eci_i + v_eci_i*dt;
v_eci = v_eci_i + a_eci  *dt;
end

== matlab function ADCS_outdated_May3/Satellite Simulator/Kinematics/Rotation Kinematics/Euler Equations ==
  data: q_i input; q output; w_i input; tor input; dt input; w output
function [q,w]  = fcn(q_i, w_i, tor, dt)

q = q_i + w_i*dt;
w = w_i + tor*dt;

== matlab function ADCS_outdated_May3/Satellite Simulator/Sensors/Sun sensor model ==
  data: sun_dir_eci input; sun_meas output; R_eci2body input; noise input; eclipse input
function sun_meas = fcn(sun_dir_eci, R_eci2body, noise, eclipse)

spx = 1;
snx = 1;
spy = 1;
sny = 1;
spz = 1;
snz = 1;

sun_meas = [spx; snx; spy; sny; spz; snz] + noise*randn([6,1]);

if(eclipse)
    sun_meas = [0;0;0;0;0;0] + noise*randn([6,1]);
end

== matlab function ADCS_outdated_May3/Satellite Simulator/Sensors/Sun sensor model1 ==
  data: R_eci2body input; w_body input; q_meas output; noise input; w_limit input
function q_meas = fcn(R_eci2body, w_body, noise, w_limit)

if norm(w_body) < w_limit
    q_meas = [1;0;0;0];
    q_meas = q_meas + noise*randn(4,1);
    q_meas = q_meas/norm(q_meas);
else
    q_meas = [1;0;0;0];
end

== matlab function ADCS_outdated_May3/Satellite Simulator/Time Model/Date2JD ==
  data: date input; JD output
function JD = fcn(date)
year   = date(1);
month  = date(2);
day    = date(3);
hour   = date(4);
minute = date(5);
second = date(6);

%replace this with real function, find text book reference from 279a
JD_Jan0_2020 = 2458848.5000;
JD = JD_Jan0_2020 + (year-2020)*365 + month*30 + day + hour/24 + minute/(24*60) + second/(24*60*60);
